simulink model "before_dac_model"  (R2026a)
settings: Solver=FixedStepAuto  StopTime=0.04  FixedStep=1e-8
settings Model: Creator=hp  LastModifiedBy=hp

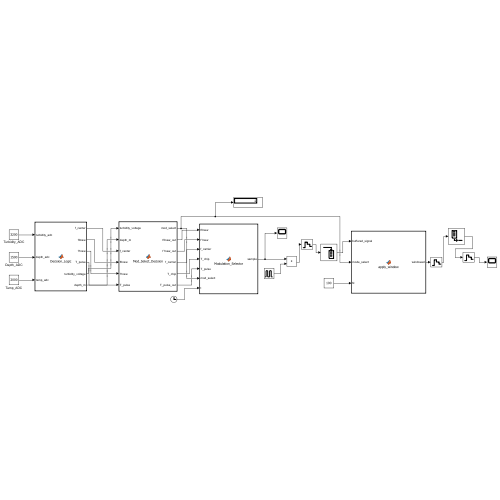
[thumbnail: Simulink's stored preview of the top-level diagram]
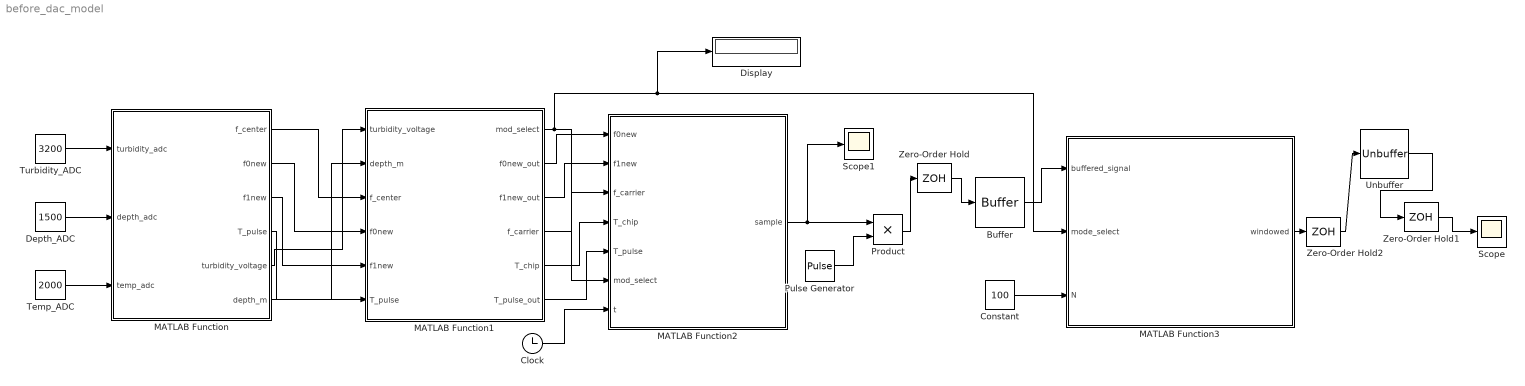
== system before_dac_model ==
  Buffer : Buffer  N=100  OutputFrames=off
  Clock : Clock
  Constant : Constant  Value=100
  Depth_ADC : Constant  Value=1500
  Display : Display
  MATLAB Function : MATLAB Function  TreatAsAtomicUnit=on
  MATLAB Function1 : MATLAB Function  TreatAsAtomicUnit=on
  MATLAB Function2 : MATLAB Function  TreatAsAtomicUnit=on
  MATLAB Function3 : MATLAB Function  TreatAsAtomicUnit=on
  Product : Product
  Pulse Generator : DiscretePulseGenerator  PulseType=Time based  Period=0.02  PulseWidth=25
  Scope : Scope
      settings: ActiveDisplayYMinimum=-1  ActiveDisplayYMaximum=1
  Scope1 : Scope
      settings: ActiveDisplayYMinimum=-1.2478348729792148  ActiveDisplayYMaximum=1.2384526558891455
  Temp_ADC : Constant  Value=2000
  Turbidity_ADC : Constant  Value=3200
  Unbuffer : Unbuffer
  Zero-Order Hold : ZeroOrderHold  SampleTime=1e-6
  Zero-Order Hold1 : ZeroOrderHold  SampleTime=-1
  Zero-Order Hold2 : ZeroOrderHold  SampleTime=1e-6
  wires:
  Turbidity_ADC/1 -> MATLAB Function/1(turbidity_adc)
  Depth_ADC/1 -> MATLAB Function/2(depth_adc)
  Temp_ADC/1 -> MATLAB Function/3(temp_adc)
  MATLAB Function/1(f_center) -> MATLAB Function1/3(f_center)
  MATLAB Function/2(f0new) -> MATLAB Function1/4(f0new)
  MATLAB Function/3(f1new) -> MATLAB Function1/5(f1new)
  MATLAB Function/4(T_pulse) -> MATLAB Function1/6(T_pulse)
  MATLAB Function/6(depth_m) -> MATLAB Function1/2(depth_m)
  MATLAB Function/5(turbidity_voltage) -> MATLAB Function1/1(turbidity_voltage)
  MATLAB Function1/2(f0new_out) -> MATLAB Function2/1(f0new)
  MATLAB Function1/1(mod_select) -> Display/1, MATLAB Function3/2(mode_select), MATLAB Function2/6(mod_select)
  MATLAB Function1/3(f1new_out) -> MATLAB Function2/2(f1new)
  MATLAB Function1/4(f_carrier) -> MATLAB Function2/3(f_carrier)
  MATLAB Function1/5(T_chip) -> MATLAB Function2/4(T_chip)
  MATLAB Function1/6(T_pulse_out) -> MATLAB Function2/5(T_pulse)
  Clock/1 -> MATLAB Function2/7(t)
  MATLAB Function2/1(sample) -> Scope1/1, Product/1
  Pulse Generator/1 -> Product/2
  Zero-Order Hold/1 -> Buffer/1
  Buffer/1 -> MATLAB Function3/1(buffered_signal)
  Constant/1 -> MATLAB Function3/3(N)
  MATLAB Function3/1(windowed) -> Zero-Order Hold2/1
  Zero-Order Hold2/1 -> Unbuffer/1
  Product/1 -> Zero-Order Hold/1
  Unbuffer/1 -> Zero-Order Hold1/1
  Zero-Order Hold1/1 -> Scope/1

== matlab function before_dac_model/MATLAB Function1 ==
  data: turbidity_voltage input; mod_select output; depth_m input; f_center input; f0new input; f1new input; T_pulse input; f0new_out output; f1new_out output; f_carrier output; T_chip output; T_pulse_out output
function [mod_select, f0new_out, f1new_out, f_carrier, T_chip, T_pulse_out] = ...
    Mod_Select_Decision(turbidity_voltage, depth_m, f_center, f0new, f1new, T_pulse)

% ---- Decide mod_select ----
if turbidity_voltage > 2.4
    mod_select = 2;      
elseif depth_m >= 30
    mod_select = 1;      
else
    mod_select = 0;     
end

% ---- Branch output params based on mod_select ----
T_pulse_out = T_pulse;   % passes through regardless of mode

if mod_select == 0 || mod_select == 1
    f0new_out = f0new;
    f1new_out = f1new;
    f_carrier = 0;       
    T_chip    = 0;       

else  % mod_select == 2
    f0new_out = 0;       
    f1new_out = 0;       
    f_carrier = f_center;
    T_chip    = T_pulse / 13;
end

end

== matlab function before_dac_model/MATLAB Function ==
  data: turbidity_adc input; f_center output; depth_adc input; temp_adc input; f0new output; f1new output; T_pulse output; turbidity_voltage output; depth_m output
function [f_center, f0new, f1new, T_pulse, turbidity_voltage, depth_m] = ...
    Decision_Logic(turbidity_adc, depth_adc, temp_adc)

turbidity_voltage = (turbidity_adc / 4095) * 3.3;
depth_voltage      = (depth_adc / 4095) * 3.3;

if turbidity_voltage <= 0.8
    f_center = 500e3;
elseif turbidity_voltage <= 2.4
    f_center = 250e3;
else
    f_center = 100e3;
end

if depth_voltage <= 0.6
    T_pulse = 1e-3;
    depth_m = 2.5;
elseif depth_voltage <= 2.0
    T_pulse = 10e-3;
    depth_m = 17.5;
else
    T_pulse = 50e-3;
    depth_m = 30;
end


T = (temp_adc / 4095) * 40;
D = depth_m;

c = 1448.96 + 4.591*T - 0.05304*T^2 + 0.0002374*T^3 ...
    + 0.0163*D + 1.675e-7*D^2 - 7.139e-13*T*D^3;

velocity  = c;
dR_target = 0.02;
B_req     = velocity / (2 * dR_target);

f0new = f_center - B_req/2;
f1new = f_center + B_req/2;

end

== matlab function before_dac_model/MATLAB Function2 ==
  data: f0new input; f1new input; f_carrier input; sample output; T_chip input; T_pulse input; mod_select input; t input
function sample = Modulation_Selector(f0new, f1new, f_carrier, T_chip, T_pulse, mod_select, t)

barker13 = [1 1 1 1 1 -1 -1 1 1 -1 1 -1 1];

if mod_select == 0
    % ---- Mode 0: LFM ----
    k = (f1new - f0new) / T_pulse;
    sample = sin(2*pi*(f0new*t + 0.5*k*t^2));

elseif mod_select == 1
    % ---- Mode 1: Geometric Sweep ----
    ratio = f1new / f0new;
    phi = (2*pi*f0new*T_pulse / log(ratio)) * (ratio^(t/T_pulse) - 1);
    sample = sin(phi);

else
    % ---- Mode 2: Phase-coded (Barker13) ----
    chip_index = mod(floor(t / T_chip), 13) + 1;
    phase_flip = barker13(chip_index);
    sample = phase_flip * sin(2*pi*f_carrier*t);
end

end

== matlab function before_dac_model/MATLAB Function3 ==
  data: buffered_signal input; windowed output; mode_select input; N input
function windowed = apply_window(buffered_signal, mode_select, N)

if mode_select == 0 || mode_select == 1

    w = blackman(N);

else

    w = rectwin(N); % Phase-coded: no window

end

windowed = buffered_signal .* w;

end
